simulink model "epc_task"  (Simulink 3.00)
settings: Solver=ode45  StartTime=0.0  StopTime=10.0  RelTol=1e-3
undefined symbols (not defined in the file): epc_uVec1, epc_uVec2, epc_yVec1, epc_yVec2
libraries: genlib x5, matrixlib x4, speclib x1
settings Model: LastModifiedBy=mertlj

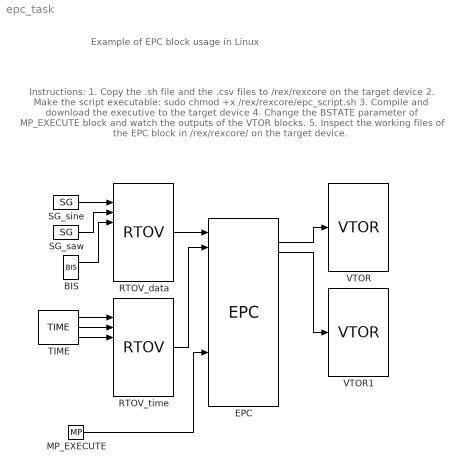
== system epc_task ==
  note: Example of EPC block usage in Linux
  note: Instructions:
      | 1. Copy the .sh file and the .csv files to /rex/rexcore on the target device
      | 2. Make the script executable: sudo chmod +x /rex/rexcore/epc_script.sh
      | 3. Compile and download the executive to the target device
      | 4. Change the BSTATE parameter of MP_EXECUTE block and watch the
      |     outputs of the VTOR blocks.
      | 5. Inspect the working files of the EPC block in /rex/rexcore/ on the target
      |     device.
  BIS : genlib/BIS  Y0=off  t1=1  t2=2  t3=3  t4=4  t5=5  t6=6  t7=7  t8=8  RPT=on
  EPC : speclib/EPC  cmd=/rex/rexcore/epc_script.sh  ifns=epc_uVec1;epc_uVec2  ofns=epc_yVec1;epc_yVec2  sl=1  ifm=10000  format=1: Space-delimited values
  MP_EXECUTE : genlib/MP  pwidth=1  BSTATE=on  RPTF=off
  RTOV_data : matrixlib/RTOV  capacity=3  offset=0  n=3
  RTOV_time : matrixlib/RTOV  capacity=3  offset=0  n=3
  SG_saw : genlib/SG  isig=3: SAWTOOTH  amp=1  freq=0.05  phase=0  ifrunit=1: Hz  iphunit=1: DEGREE
  SG_sine : genlib/SG  isig=1: SINE  amp=1  freq=0.01  phase=0  ifrunit=1: Hz  iphunit=1: DEGREE
  TIME : genlib/TIME  tz=1: Local time
  VTOR : matrixlib/VTOR  n=5  offset=0
  VTOR1 : matrixlib/VTOR  n=3  offset=0
  wires:
  BIS/1 -> RTOV_data/4
  EPC/1 -> VTOR/1
  EPC/2 -> VTOR1/1
  MP_EXECUTE/1 -> EPC/9
  RTOV_data/1 -> EPC/1
  RTOV_time/1 -> EPC/2
  SG_saw/1 -> RTOV_data/3
  SG_sine/1 -> RTOV_data/2
  TIME/1 -> RTOV_time/2
  TIME/2 -> RTOV_time/3
  TIME/3 -> RTOV_time/4
